simulink model "serie_b"  (R2019a)
settings: Solver=VariableStepAuto  StartTime=0.0  StopTime=10.0  RelTol=1e-3
undefined symbols (not defined in the file): Tl, Va, Vf
libraries: powerlib x4
settings Model: Creator=azizi  LastModifiedBy=azizi

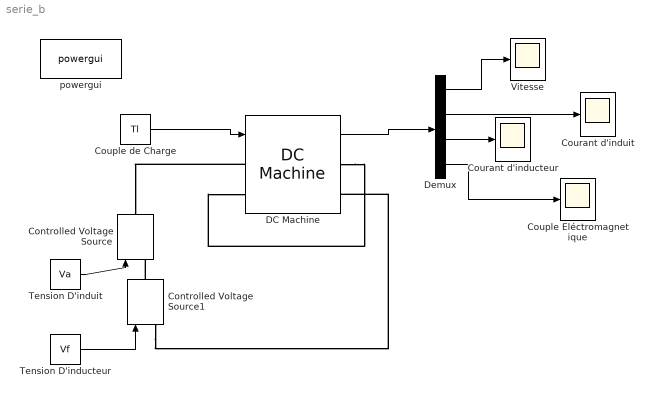
== system serie_b ==
  Controlled Voltage Source : powerlib/Electrical Sources/Controlled Voltage Source  Initialize=on  Source_Type=AC  Amplitude=0  Phase=0  Frequency=0  Measurements=None
      settings: SourceProductName=Simscape Electrical
  Controlled Voltage Source1 : powerlib/Electrical Sources/Controlled Voltage Source  Initialize=on  Source_Type=AC  Amplitude=0  Phase=0  Frequency=0  Measurements=None
      settings: SourceProductName=Simscape Electrical
  Couple Eléctromagnetique : Scope
  Couple de Charge : Constant  Value=Tl
  Courant d'inducteur : Scope
  Courant d'induit : Scope
  DC Machine : powerlib/Machines/DC Machine  PresetModel=No  MechanicalLoad=Torque TL  FieldType=Wound  ShowDetailedParameters=on  MeasurementBus=off  RLa="[ 1.5  0.12]"  RLf="[ 0.7  0.03]"  Laf=0.0675  MachineConstant=Torque constant (N.m/A)  Ke=1.8  Kt=1.8  J=0.02365  Bm=2.5e-3  Tf=0  w0=0  Ifinit=0  TsPowergui=0  TsBlock=-1
      settings: SourceProductName=Simscape Electrical
  Demux : Demux
  Tension D'inducteur : Constant  Value=Vf
  Tension D'induit : Constant  Value=Va
  "Vitesse " : Scope
  powergui : powerlib/powergui  Priority=1  SimulationMode=Continuous  SampleTime=50e-6  frequency=60  Iterations=50  frequencyindice=0  Pbase=100e6  ErrMax=1e-4  UnitsV=kV  UnitsW=MW  buscounter=0  FunctionMessages=off  echomessages=off  EnableUseOfTLC=off  CurrentSourceSwitches=off  DisableSnubberDevices=off  DisableRonSwitches=off  DisableVfSwitches=off  DisplayEquations=off  AutomaticDiscreteSolvers=off  SolverType=Tustin/Backward Euler (TBE)  Interpol=off  ExternalGateDelay=off  methode=off  Ts=100  x0status=blocks  SPID=on  SwTol=0  HookPort=off  NonlinearTolerance=0  nMaxIteration=15  ContinueOnMaxIteration=off  RestoreLinks=warning  ResistiveCurrentMeasurement=off  Frange=[0:2:500]  Ylog=off  Xlog=on  ShowGrid=off  save=off  variable=ZData  structure=0  ZoomFFT=off  StartTime=0.0  cycles=1  DisplayStyle=1  fundamental=60  FreqAxis=off  MaxFrequency=1000  frequencyindicesteady=1  RmsSteady=1  display=off
      settings: SourceProductName=Simscape Electrical
  wires:
  Couple de Charge/1 -> DC Machine/1
  Tension D'induit/1 -> Controlled Voltage Source/1
  DC Machine/1 -> Demux/1
  Demux/1 -> "Vitesse "/1
  Demux/2 -> Courant d'induit/1
  Demux/3 -> Courant d'inducteur/1
  Demux/4 -> Couple Eléctromagnetique/1
  Tension D'inducteur/1 -> Controlled Voltage Source1/1
  connections:
  DC Machine/LConn1 -- Controlled Voltage Source/RConn1
  DC Machine/RConn1 -- DC Machine/LConn2
  Controlled Voltage Source1/RConn1 -- Controlled Voltage Source/LConn1
  Controlled Voltage Source1/LConn1 -- DC Machine/RConn2
